simulink model "Electromagetic_Energy_Harvesting"  (R2021a)
settings: Solver=ode23tb  StartTime=0.0  StopTime=1  RelTol=1e-3  EnableMultiTasking=on
libraries: spsSeriesRLCBranchLib x9, spsDiodeLib x4, simulink x2, spsMosfetLib x2, spsControlledVoltageSourceLib x1, spsCurrentMeasurementLib x1, spsVoltageMeasurementLib x1, spspowerguiLib x1
settings Model: Creator=home  LastModifiedBy=USER
settings SolverCC: ZeroCrossAlgorithm=Adaptive  AlgebraicLoopSolver=TrustRegion
settings DataIOCC: LimitDataPoints=on  SaveFormat=Array  SignalLoggingSaveFormat=ModelDataLogs  ReturnWorkspaceOutputs=off
settings OptimizationCC: ExpressionDepthLimit=2147483647  InitFltsAndDblsToZero=on  LifeSpan=inf
settings DebuggingCC: UnderspecifiedInitializationDetection=Classic  MergeDetectMultiDrivingBlocksExec=none  SolverPrmCheckMsg=warning  FcnCallInpInsideContextMsg=warning  StateNameClashWarn=warning  SFUnexpectedBacktrackingDiag=warning  SFNoUnconditionalDefaultTransitionDiag=warning  SFExecutionAtInitializationDiag=none  SFMachineParentedDataDiag=warning  ArithmeticOperatorsInVariantConditions=warning
settings HardwareCC: ProdBitPerPointer=32  ProdBitPerSizeT=32  ProdBitPerPtrDiffT=32  ProdLargestAtomicFloat=None  ProdIntDivRoundTo=Undefined  ProdEndianess=Unspecified  ProdWordSize=32  ProdHWDeviceType=32-bit Generic
settings ModelReferenceCC: PropagateSignalLabelsOutOfModel=off
settings SFSimCC: SimUseLocalCustomCode=off  SimParseCustomCode=off  CustomCodeUndefinedFunction=UseInterfaceOnly
settings RTWCC: RTWUseLocalCustomCode=off
settings CodeAppCC: StateflowObjectComments=on
settings GRTTargetCC: TargetLangStandard=C89/C90 (ANSI)  CombineOutputUpdateFcns=off  GRTInterface=on
settings ConfigComp: CovMetricSettings=dw  CovSaveCumulativeToWorkspaceVar=on  CovSaveSingleToWorkspaceVar=on  CovExternalEMLEnable=off

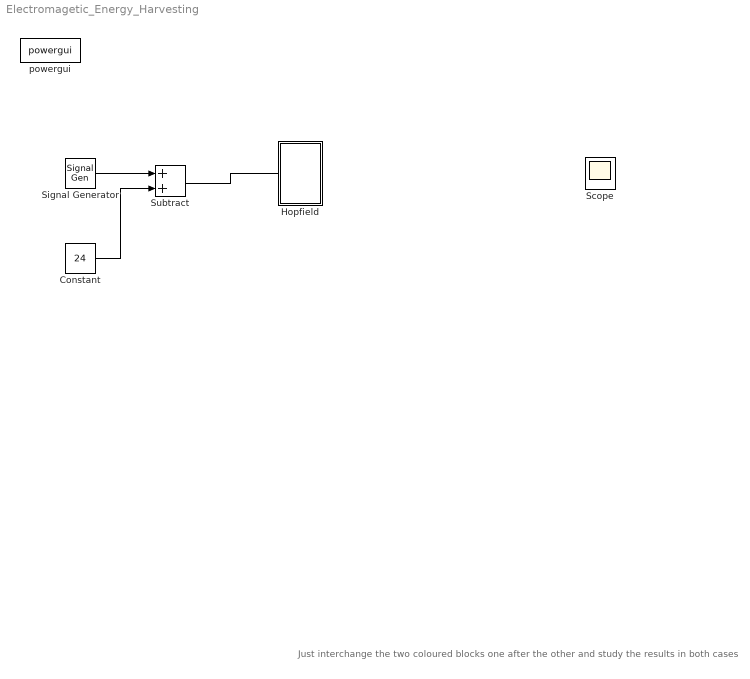
== system Electromagetic_Energy_Harvesting ==
  note: Just interchange the two coloured blocks one after the other
      | and study the results in both cases
  Constant : Constant  Value=24
  Hopfield : Subsystem
  Scope : Scope
  Signal Generator : SignalGenerator  WaveForm=square  Amplitude=15  Frequency=3
  Subtract : Sum
  powergui : spspowerguiLib/powergui  SimulationMode=Discrete  SampleTime=5e-6  frequency=60  Iterations=50  frequencyindice=0  Pbase=100e6  ErrMax=1e-4  UnitsV=kV  UnitsW=MW  buscounter=0  FunctionMessages=off  echomessages=off  EnableUseOfTLC=off  CurrentSourceSwitches=off  DisableSnubberDevices=off  DisableRonSwitches=off  DisableVfSwitches=off  DisplayEquations=off  AutomaticDiscreteSolvers=off  SolverType=Tustin/Backward Euler (TBE)  Interpol=off  ExternalGateDelay=off  methode=off  Ts=0  x0status=blocks  SPID=off  SwTol=0  HookPort=off  NonlinearTolerance=1e-4  nMaxIteration=100  ContinueOnMaxIteration=off  RestoreLinks=warning  ResistiveCurrentMeasurement=off  Frange=[0:2:500]  Ylog=off  Xlog=on  ShowGrid=off  save=off  variable=ZData  structure=0  ZoomFFT=on  StartTime=0.0  cycles=1  DisplayStyle=1  fundamental=60  FreqAxis=off  MaxFrequency=1000  frequencyindicesteady=1  RmsSteady=1  display=off
  wires:
  ? -> Scope/1
  Signal Generator/1 -> Subtract/1
  Constant/1 -> Subtract/2
  Subtract/1 -> ?

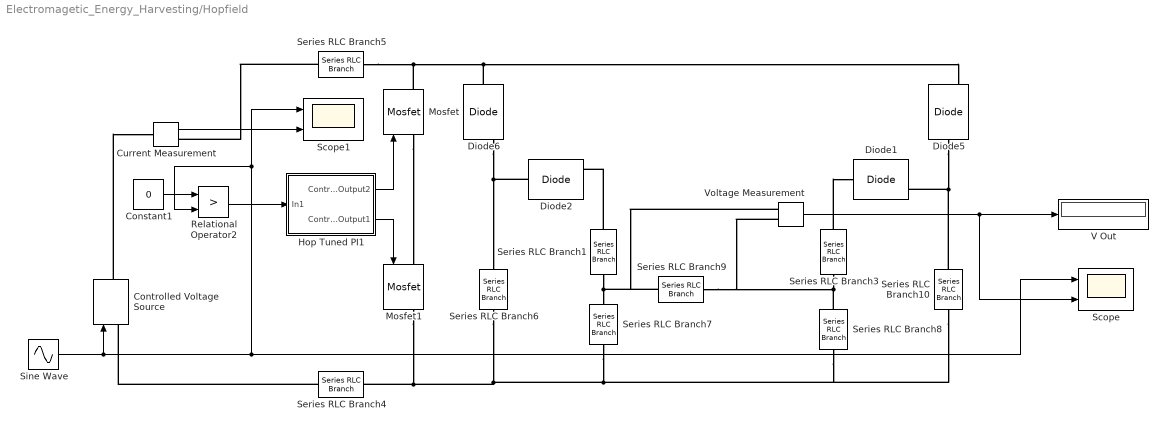
== system Electromagetic_Energy_Harvesting/Hopfield ==
  Constant1 : Constant  Value=0
  Controlled Voltage Source : spsControlledVoltageSourceLib/Controlled Voltage Source  Initialize=on  Source_Type=AC  Amplitude=0  Phase=0  Frequency=0  Measurements=None
  Current Measurement : spsCurrentMeasurementLib/Current Measurement  PhasorSimulation=off  OutputType=Complex  PSBequivalent=0
  Diode{1..2,5..6} (4 alike) : spsDiodeLib/Diode  Ron=0.001  Lon=0  Vf=0.8  IC=0  UseSnubber=off  Rs=500  Cs=250e-9  Measurements=on
  Hop Tuned PI1 : Subsystem
  Mosfet : spsMosfetLib/Mosfet  Ron=0.01  Lon=0  Rd=0.01  Vfd=0  IC=0  Rs=1e5  Cs=inf  Measurements=on
  Mosfet1 : spsMosfetLib/Mosfet  Ron=0.01  Lon=0  Rd=0.01  Vfd=0  IC=0  Rs=1e5  Cs=inf  Measurements=on
  Relational Operator2 : RelationalOperator  Operator=>  OutDataTypeStr=boolean  RndMeth=Nearest
  Scope : Scope  NumInputPorts=2
  Scope1 : Scope  NumInputPorts=2
  Series RLC Branch{1,3..5} (4 alike) : spsSeriesRLCBranchLib/Series RLC Branch  LConnTagsString=__new0  RConnTagsString=__new0  BranchType=RL  Resistance=0.001  Inductance=1e-3  SetiL0=off  InitialCurrent=0  Capacitance=1e-6  Setx0=off  InitialVoltage=0  Measurements=None
  Series RLC Branch10 : spsSeriesRLCBranchLib/Series RLC Branch  LConnTagsString=__new0  RConnTagsString=__new0  BranchType=C  Resistance=1  Inductance=50e-6  SetiL0=off  InitialCurrent=0  Capacitance=250e-6  Setx0=off  InitialVoltage=0  Measurements=None
  Series RLC Branch6 : spsSeriesRLCBranchLib/Series RLC Branch  LConnTagsString=__new0  RConnTagsString=__new0  BranchType=C  Resistance=1  Inductance=50e-6  SetiL0=off  InitialCurrent=0  Capacitance=250e-6  Setx0=off  InitialVoltage=0  Measurements=None
  Series RLC Branch7 : spsSeriesRLCBranchLib/Series RLC Branch  LConnTagsString=__new0  RConnTagsString=__new0  BranchType=C  Resistance=1  Inductance=50e-6  SetiL0=off  InitialCurrent=0  Capacitance=2500e-6  Setx0=off  InitialVoltage=0  Measurements=None
  Series RLC Branch8 : spsSeriesRLCBranchLib/Series RLC Branch  LConnTagsString=__new0  RConnTagsString=__new0  BranchType=C  Resistance=1  Inductance=50e-6  SetiL0=off  InitialCurrent=0  Capacitance=2500e-6  Setx0=off  InitialVoltage=0  Measurements=None
  Series RLC Branch9 : spsSeriesRLCBranchLib/Series RLC Branch  LConnTagsString=__new0  RConnTagsString=__new0  BranchType=R  Resistance=100  Inductance=1e-3  SetiL0=off  InitialCurrent=0  Capacitance=1e-6  Setx0=off  InitialVoltage=0  Measurements=None
  Sine Wave : Sin  Amplitude=24  Frequency=2*(22/7)*100  SampleTime=0
  V Out : Display
  Voltage Measurement : spsVoltageMeasurementLib/Voltage Measurement  PhasorSimulation=off  OutputType=Complex  PSBequivalent=0
  wires:
  Voltage Measurement/1 -> Scope/2, V Out/1
  Hop Tuned PI1/1(Control Output2) -> Mosfet/1
  Sine Wave/1 -> Scope/1, Scope1/1, Relational Operator2/2, Controlled Voltage Source/1
  Current Measurement/1 -> Scope1/2
  Constant1/1 -> Relational Operator2/1
  Relational Operator2/1 -> Hop Tuned PI1/1(In1)
  Hop Tuned PI1/2(Control Output1) -> Mosfet1/1
  connections:
  Controlled Voltage Source/RConn1 -- Current Measurement/LConn1
  Series RLC Branch5/RConn1 -- Current Measurement/RConn1
  Series RLC Branch4/LConn1 -- Controlled Voltage Source/LConn1
  Series RLC Branch5/LConn1 -- Diode5/RConn1 -- Diode6/LConn1 -- Mosfet/RConn1
  Mosfet1/RConn1 -- Series RLC Branch8/LConn1 -- Series RLC Branch10/RConn1 -- Series RLC Branch7/RConn1 -- Series RLC Branch6/RConn1 -- Series RLC Branch4/RConn1
  Mosfet/LConn1 -- Mosfet1/LConn1
  Diode6/RConn1 -- Diode2/LConn1 -- Series RLC Branch6/LConn1
  Series RLC Branch1/LConn1 -- Diode2/RConn1
  Diode5/LConn1 -- Series RLC Branch10/LConn1 -- Diode1/RConn1
  Series RLC Branch3/LConn1 -- Diode1/LConn1
  Series RLC Branch1/RConn1 -- Voltage Measurement/LConn1 -- Series RLC Branch9/RConn1 -- Series RLC Branch7/LConn1
  Series RLC Branch3/RConn1 -- Series RLC Branch8/RConn1 -- Voltage Measurement/LConn2 -- Series RLC Branch9/LConn1

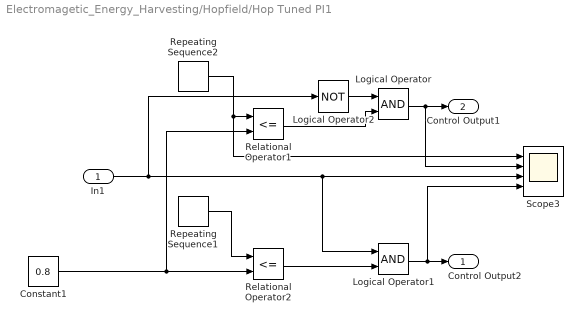
== system Electromagetic_Energy_Harvesting/Hopfield/Hop Tuned PI1 ==
  In1 : Inport
  Constant1 : Constant  Value=0.8
  Logical Operator : Logic  AllPortsSameDT=off  OutDataTypeStr=boolean
  Logical Operator1 : Logic  AllPortsSameDT=off  OutDataTypeStr=boolean
  Logical Operator2 : Logic  Operator=NOT  AllPortsSameDT=off  OutDataTypeStr=boolean
  Relational Operator1 : RelationalOperator  Operator=<=  OutDataTypeStr=boolean  RndMeth=Nearest
  Relational Operator2 : RelationalOperator  Operator=<=  OutDataTypeStr=boolean  RndMeth=Nearest
  Repeating Sequence1 : simulink/Sources/Repeating Sequence  rep_seq_t="[0 1/(40e3)  1/(20e3)]"  rep_seq_y="[1 0  1 ]"
  Repeating Sequence2 : simulink/Sources/Repeating Sequence  rep_seq_t="[0 1/(40e3)  1/(20e3)]"  rep_seq_y="[0  1 0 ]"
  Scope3 : Scope  NumInputPorts=4
  Control Output2 : Outport
  Control Output1 : Outport  Port=2
  wires:
  Relational Operator1/1 -> Logical Operator/2
  Repeating Sequence2/1 -> Scope3/1, Relational Operator1/1
  Constant1/1 -> Relational Operator1/2, Relational Operator2/2
  Repeating Sequence1/1 -> Relational Operator2/1
  Relational Operator2/1 -> Logical Operator1/2
  In1/1 -> Logical Operator1/1, Scope3/3, Logical Operator2/1
  Logical Operator2/1 -> Logical Operator/1
  Logical Operator/1 -> Scope3/2, Control Output1/1
  Logical Operator1/1 -> Scope3/4, Control Output2/1
